simulink model "RE35"  (Simulink 10.1)
settings: Solver=VariableStepAuto  StartTime=0.0  StopTime=0.05  RelTol=1e-3
values from neighbouring files (symbols this model uses):
  J = 6.81e-6    (= 6.81e-06)    [DC_contr_ZN.m]    (also in DC_mot_TF.m; RE_35.m)
  K_b = 0.0388    [DC_contr_ZN.m]    (also in DC_mot_TF.m; Maxon_Control_BD.m = 0.0388182788029; RE_35.m)
  K_f = 6.33e-6    (= 6.33e-06)    [DC_contr_ZN.m]    (also in DC_mot_TF.m; Kf.m = 6.33589917605e-06; Maxon_Control_BD.m = 4.80152536515e-06; RE_35.m)
  K_m = 0.0389    [DC_contr_ZN.m]    (also in DC_mot_TF.m; Kf.m; Maxon_Control_BD.m; RE_35.m)
  L = 0.34e-3    (= 0.00034)    [DC_contr_ZN.m]    (also in DC_mot_TF.m; RE_35.m)
  R = 1.2    [DC_contr_ZN.m]    (also in DC_mot_TF.m; RE_35.m)
  T_nom = 0.0972    [DC_contr_ZN.m]    (also in DC_mot_TF.m; Maxon_Control_BD.m = 0.101; RE_35.m)
  U_nom = 30    [RE_35.m]
settings Model: Creator=manfred  LastModifiedBy=manfred
settings DataIOCC: SaveFormat=Dataset  ReturnWorkspaceOutputs=on
settings OptimizationCC: LifeSpan=auto
settings DebuggingCC: UnderspecifiedInitializationDetection=Simplified  MergeDetectMultiDrivingBlocksExec=error  SFUnexpectedBacktrackingDiag=error  SFNoUnconditionalDefaultTransitionDiag=error  SFExecutionAtInitializationDiag=warning  ArithmeticOperatorsInVariantConditions=error
settings HardwareCC: ProdBitPerPointer=64  ProdBitPerSizeT=64  ProdBitPerPtrDiffT=64  ProdLargestAtomicFloat=Float  ProdIntDivRoundTo=Zero  ProdEndianess=LittleEndian  ProdWordSize=64  ProdHWDeviceType=Intel->x86-64 (Windows64)
settings ModelReferenceCC: PropagateSignalLabelsOutOfModel=on
settings SFSimCC: SimUseLocalCustomCode=on  CustomCodeUndefinedFunction=FilterOut
settings RTWCC: RTWUseLocalCustomCode=on
settings CodeAppCC: StateflowObjectComments=off
settings GRTTargetCC: TargetLangStandard=C99 (ISO)  CombineOutputUpdateFcns=on  GRTInterface=off
settings ConfigComp: CovMetricSettings=dwe  CovHtmlReporting=off  CovSaveCumulativeToWorkspaceVar=off  CovSaveSingleToWorkspaceVar=off  CovExternalEMLEnable=on

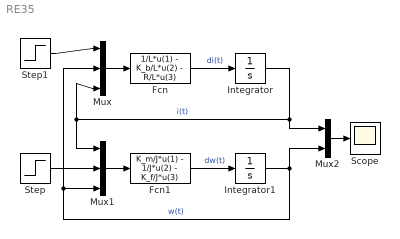
== system RE35 ==
  Fcn : Fcn  Expr=1/L*u(1) - K_b/L*u(2) - R/L*u(3)
  Fcn1 : Fcn  Expr=K_m/J*u(1) - 1/J*u(2) - K_f/J*u(3)
  Integrator : Integrator
  Integrator1 : Integrator
  Mux : Mux  Inputs=3
  Mux1 : Mux  Inputs=3
  Mux2 : Mux  Inputs=2
  Scope : Scope
  Step : Step  Time=0.02  After=T_nom  SampleTime=0
  Step1 : Step  Time=0  After=U_nom  SampleTime=0
  wires:
  Fcn/1 -> Integrator/1  "di(t)"
  Mux/1 -> Fcn/1
  Integrator/1 -> Mux2/1, Mux1/1, Mux/3  "i(t)"
  Integrator1/1 -> Mux2/2, Mux1/3, Mux/2  "w(t)"
  Mux1/1 -> Fcn1/1
  Fcn1/1 -> Integrator1/1  "dw(t)"
  Step/1 -> Mux1/2
  Step1/1 -> Mux/1
  Mux2/1 -> Scope/1
